simulink model "tesdd"  (R2012b)
settings: Solver=ode45  StartTime=0.0  StopTime=25000  RelTol=1e-3
undefined symbols (not defined in the file or in its folder): pfb_coeff_gen_calc, sfp
undefined symbols (not defined in the file): SL, transtable
libraries: xbsIndex_r4 x5296, casper_library_misc x104, casper_library_delays x24, xps_library x14, maddogLibrary x4, simulink x2
(part 37 of 52)

== system tesdd/FRD2/DFT/costable/mem ==
  note: Undo data manipulation on way in and redo on way out for simulated data
  note: Undo address
      | manipulation for
      | simulated data
  In1 : Inport
  In2 : Inport  Port=2
  In3 : Inport  Port=3
  Disregard Subsystem : xbsIndex_r4/Disregard Subsystem  Tag=discardX  block_type=disregard
  calc_add : Subsystem  mask{data_width=16, addr_width=11, sample_rate=sample_rate}
      mask prompts: data_width "data width"; addr_width "address width"; sample_rate "sample rate"
  ram : xbsIndex_r4/Single Port RAM  depth=2^addr_width  initVector=init_vals  distributed_mem=Block RAM  write_mode=Read After Write  rst=off  init_reg=0  en=off  latency=1  dbl_ovrd=off  optimize=Area  block_type=spram
  sim_addr : xbsIndex_r4/Gateway In  gui_display_data_type=Fixed-point  arith_type=Unsigned  n_bits=addr_width  bin_pt=0  preci_type=Single  exp_width=8  frac_width=24  quantization=Truncate  overflow=Wrap  period=sample_rate  dbl_ovrd=off  timing_constraint=None  locs_specified=off  LOCs={}  UseAsADC=off  ADCChannel='1'  inherit_from_input=off  hdl_port=on  block_type=gatewayin
      settings: infoedit="Gateway in block.  Converts inputs of type Simulink integer, double and fixed point to  Xilinx fixed point type.<br><br>Hardware notes:  In hardware these blocks become top level input ports."  xl_area=[0, 0, 0, 0, 0, 0, 0]  sginterface={'Nallatech'=>{'xdspkit'=>{'non_memory_mapped_port'=>'sim_addr'}},'Xilinx'=>{'jtaghwcosim'=>{'non_memory_mapped_port'=>'sim_addr'},'xdspkit'=>{'non_memory_mapped_port'=>'sim_addr'}}}
  sim_data_in : xbsIndex_r4/Gateway In  gui_display_data_type=Fixed-point  arith_type=Unsigned  n_bits=16  bin_pt=14  preci_type=Single  exp_width=8  frac_width=24  quantization=Truncate  overflow=Wrap  period=sample_rate  dbl_ovrd=off  timing_constraint=None  locs_specified=off  LOCs={}  UseAsADC=off  ADCChannel='1'  inherit_from_input=off  hdl_port=on  block_type=gatewayin
      settings: xl_area=[0, 0, 0, 0, 0, 0, 0]  sginterface={'Nallatech'=>{'xdspkit'=>{'non_memory_mapped_port'=>'sim_data_in'}},'Xilinx'=>{'jtaghwcosim'=>{'non_memory_mapped_port'=>'sim_data_in'},'xdspkit'=>{'non_memory_mapped_port'=>'sim_data_in'}}}
  sim_data_out : xbsIndex_r4/Gateway Out  inherit_from_input=off  hdl_port=on  timing_constraint=None  locs_specified=off  LOCs={'B21','B22','A22','B23','B19','C19','A20','A21','A23','B24','A24','A25','E18','D18','C18','B18'}  UseAsDAC=off  DACChannel='1'  block_type=gatewayout
      settings: infoedit="Gateway out block.  Converts Xilinx fixed point inputs into ouputs of type Simulink integer, double, or fixed point.<P><P>Hardware notes:  In hardware these blocks become top level output ports or are discarded, depending on how they are configured."  xl_area=[0, 0, 0, 0, 0, 0, 0]  sginterface={'Nallatech'=>{'xdspkit'=>{'non_memory_mapped_port'=>'sim_data_out'}},'Xilinx'=>{'jtaghwcosim'=>{'non_memory_mapped_port'=>'sim_data_out'},'xdspkit'=>{'non_memory_mapped_port'=>'sim_data_out'}}}
  sim_munge_in : Subsystem  AncestorBlock=casper_library_flow_control/munge  mask(munge){divisions=1, div_size=16, order=[0], arith_type_out=Signed  (2's comp), bin_pt_out=14}
      mask prompts: divisions "Number of divisions"; div_size "Division size (bits)"; order "Division packing order"; arith_type_out "Output arithmetic type"; bin_pt_out "Output binary point"
      mask help: Splits an input bus into the specified number of divisions and then recombines them in the order specified (most significant division = 0,least = number divisions-1)
      mask init:
      | munge_init(gcb, ...
      |     'divisions', divisions, ...
      |     'div_size', div_size, ...
      |     'order', order, ...
      |     'arith_type_out', arith_type_out, ...
      |     'bin_pt_out', bin_pt_out);
      settings: AttributesFormatString=|
      | split:16
      | join:0
      | Signed  (2's comp) [16,14]
      mask TypeOptions arith_type_out: Unsigned | Signed  (2's comp) | Floating-point
  sim_munge_out : Subsystem  AncestorBlock=casper_library_flow_control/munge  mask(munge){divisions=1, div_size=16, order=[0], arith_type_out=Unsigned, bin_pt_out=14}
      mask prompts: divisions "Number of divisions"; div_size "Division size (bits)"; order "Division packing order"; arith_type_out "Output arithmetic type"; bin_pt_out "Output binary point"
      mask help: Splits an input bus into the specified number of divisions and then recombines them in the order specified (most significant division = 0,least = number divisions-1)
      mask init:
      | munge_init(gcb, ...
      |     'divisions', divisions, ...
      |     'div_size', div_size, ...
      |     'order', order, ...
      |     'arith_type_out', arith_type_out, ...
      |     'bin_pt_out', bin_pt_out);
      settings: AttributesFormatString=|
      | split:16
      | join:0
      | Unsigned [16,14]
      mask TypeOptions arith_type_out: Unsigned | Signed  (2's comp) | Floating-point
  sim_we : xbsIndex_r4/Gateway In  gui_display_data_type=Fixed-point  arith_type=Boolean  n_bits=1  bin_pt=0  preci_type=Single  exp_width=8  frac_width=24  quantization=Truncate  overflow=Wrap  period=sample_rate  dbl_ovrd=off  timing_constraint=None  locs_specified=off  LOCs={}  UseAsADC=off  ADCChannel='1'  inherit_from_input=off  hdl_port=on  block_type=gatewayin
      settings: infoedit="Gateway in block.  Converts inputs of type Simulink integer, double and fixed point to  Xilinx fixed point type.<br><br>Hardware notes:  In hardware these blocks become top level input ports."  xl_area=[0, 0, 0, 0, 0, 0, 0]  sginterface={'Nallatech'=>{'xdspkit'=>{'non_memory_mapped_port'=>'sim_we'}},'Xilinx'=>{'jtaghwcosim'=>{'non_memory_mapped_port'=>'sim_we'},'xdspkit'=>{'non_memory_mapped_port'=>'sim_we'}}}
  Out1 : Outport
  wires:
  calc_add/1(out) -> ram/1
  sim_munge_out/1(dout) -> sim_data_out/1
  In1/1 -> sim_addr/1
  In2/1 -> sim_data_in/1
  sim_data_out/1 -> Out1/1
  In3/1 -> sim_we/1
  sim_addr/1 -> calc_add/1(in)
  sim_data_in/1 -> sim_munge_in/1(din)
  sim_we/1 -> ram/3
  ram/1 -> sim_munge_out/1(din)
  sim_munge_in/1(dout) -> ram/2

== system tesdd/FRD2/DFT/costable/munge_in ==
  din : Inport
  reinterpret_out : xbsIndex_r4/Reinterpret  force_arith_type=on  arith_type=Unsigned  force_bin_pt=on  bin_pt=14  block_type=reinterpret
  dout : Outport
  wires:
  reinterpret_out/1 -> dout/1
  din/1 -> reinterpret_out/1

== system tesdd/FRD2/DFT/costable/munge_out ==
  din : Inport
  reinterpret_out : xbsIndex_r4/Reinterpret  force_arith_type=on  arith_type="Signed  (2's comp)"  force_bin_pt=on  bin_pt=14  block_type=reinterpret
  dout : Outport
  wires:
  reinterpret_out/1 -> dout/1
  din/1 -> reinterpret_out/1

== system tesdd/FRD2/DFT/sintable/calc_add ==
  note: Use behavioural HDL
      | so that gets optimised
      | to minimum logic
  note: If reading/writing words
      | smaller than 32 bits,
      | change address so
      | that addressing is
      | big endian instead of
      | little, otherwise
      | pass through
  in : Inport
  add_sub : xbsIndex_r4/AddSub  mode=Subtraction  use_carryin=off  use_carryout=off  en=off  latency=0  precision=User Defined  arith_type=Unsigned  n_bits=max(1, log2(32/data_width))  bin_pt=0  quantization=Truncate  overflow=Wrap  dbl_ovrd=off  use_behavioral_HDL=on  hw_selection=Fabric  pipelined=off  block_type=addsub
  concat : xbsIndex_r4/Concat  num_inputs=2  dbl_ovrd=off  block_type=concat
  const : xbsIndex_r4/Constant  const=max(0, 32/data_width-1)  gui_display_data_type=Fixed-point  arith_type=Unsigned  n_bits=max(1, log2(32/data_width))  bin_pt=0  preci_type=Single  exp_width=8  frac_width=24  explicit_period=on  period=sample_rate  equ=P=C  opselect=C  inp2=PCIN>>17  opr=+  inp1=P  carry=CIN  dbl_ovrd=off  block_type=constant
      settings: block_version=11.4
  convert_addr : xbsIndex_r4/Convert  gui_display_data_type=Fixed-point  arith_type=Unsigned  n_bits=addr_width  bin_pt=0  float_type=Single  exp_bits=8  fraction_bits=24  quantization=Truncate  overflow=Wrap  en=off  latency=0  dbl_ovrd=off  pipeline=off  block_type=convert
      settings: xl_area=[0, 0, 0, 0, 0, 0, 0]
  lsw : xbsIndex_r4/Slice  nbits=max(1, log2(32/data_width))  boolean_output=off  mode=Lower Bit Location + Width  bit1=0  base1=MSB of Input  bit0=0  base0=LSB of Input  dbl_ovrd=off  block_type=slice
  manipulate : xbsIndex_r4/Constant  const=min(1, floor(32/data_width) - 1)  gui_display_data_type=Fixed-point  arith_type=Unsigned  n_bits=1  bin_pt=0  preci_type=Single  exp_width=8  frac_width=24  explicit_period=on  period=sample_rate  equ=P=C  opselect=C  inp2=PCIN>>17  opr=+  inp1=P  carry=CIN  dbl_ovrd=off  block_type=constant
      settings: block_version=11.4
  msw : xbsIndex_r4/Slice  nbits=addr_width - max(1, log2(32/data_width))  boolean_output=off  mode=Upper Bit Location + Width  bit1=0  base1=MSB of Input  bit0=0  base0=LSB of Input  dbl_ovrd=off  block_type=slice
  mux : xbsIndex_r4/Mux  inputs=2  en=off  latency=0  precision=Full  arith_type=Unsigned  n_bits=16  bin_pt=14  quantization=Truncate  overflow=Wrap  dbl_ovrd=off  block_type=mux
      settings: block_version=11.4
  out : Outport
  wires:
  convert_addr/1 -> mux/2, msw/1, lsw/1
  const/1 -> add_sub/1
  lsw/1 -> add_sub/2
  mux/1 -> out/1
  manipulate/1 -> mux/1
  concat/1 -> mux/3
  msw/1 -> concat/1
  add_sub/1 -> concat/2
  in/1 -> convert_addr/1

== system tesdd/FRD2/DFT/sintable/mem ==
  note: Undo data manipulation on way in and redo on way out for simulated data
  note: Undo address
      | manipulation for
      | simulated data
  In1 : Inport
  In2 : Inport  Port=2
  In3 : Inport  Port=3
  Disregard Subsystem : xbsIndex_r4/Disregard Subsystem  Tag=discardX  block_type=disregard
  calc_add : Subsystem  mask{data_width=16, addr_width=11, sample_rate=sample_rate}
      mask prompts: data_width "data width"; addr_width "address width"; sample_rate "sample rate"
  ram : xbsIndex_r4/Single Port RAM  depth=2^addr_width  initVector=init_vals  distributed_mem=Block RAM  write_mode=Read After Write  rst=off  init_reg=0  en=off  latency=1  dbl_ovrd=off  optimize=Area  block_type=spram
  sim_addr : xbsIndex_r4/Gateway In  gui_display_data_type=Fixed-point  arith_type=Unsigned  n_bits=addr_width  bin_pt=0  preci_type=Single  exp_width=8  frac_width=24  quantization=Truncate  overflow=Wrap  period=sample_rate  dbl_ovrd=off  timing_constraint=None  locs_specified=off  LOCs={}  UseAsADC=off  ADCChannel='1'  inherit_from_input=off  hdl_port=on  block_type=gatewayin
      settings: infoedit="Gateway in block.  Converts inputs of type Simulink integer, double and fixed point to  Xilinx fixed point type.<br><br>Hardware notes:  In hardware these blocks become top level input ports."  xl_area=[0, 0, 0, 0, 0, 0, 0]  sginterface={'Nallatech'=>{'xdspkit'=>{'non_memory_mapped_port'=>'sim_addr'}},'Xilinx'=>{'jtaghwcosim'=>{'non_memory_mapped_port'=>'sim_addr'},'xdspkit'=>{'non_memory_mapped_port'=>'sim_addr'}}}
  sim_data_in : xbsIndex_r4/Gateway In  gui_display_data_type=Fixed-point  arith_type=Unsigned  n_bits=16  bin_pt=14  preci_type=Single  exp_width=8  frac_width=24  quantization=Truncate  overflow=Wrap  period=sample_rate  dbl_ovrd=off  timing_constraint=None  locs_specified=off  LOCs={}  UseAsADC=off  ADCChannel='1'  inherit_from_input=off  hdl_port=on  block_type=gatewayin
      settings: xl_area=[0, 0, 0, 0, 0, 0, 0]  sginterface={'Nallatech'=>{'xdspkit'=>{'non_memory_mapped_port'=>'sim_data_in'}},'Xilinx'=>{'jtaghwcosim'=>{'non_memory_mapped_port'=>'sim_data_in'},'xdspkit'=>{'non_memory_mapped_port'=>'sim_data_in'}}}
  sim_data_out : xbsIndex_r4/Gateway Out  inherit_from_input=off  hdl_port=on  timing_constraint=None  locs_specified=off  LOCs={'B21','B22','A22','B23','B19','C19','A20','A21','A23','B24','A24','A25','E18','D18','C18','B18'}  UseAsDAC=off  DACChannel='1'  block_type=gatewayout
      settings: infoedit="Gateway out block.  Converts Xilinx fixed point inputs into ouputs of type Simulink integer, double, or fixed point.<P><P>Hardware notes:  In hardware these blocks become top level output ports or are discarded, depending on how they are configured."  xl_area=[0, 0, 0, 0, 0, 0, 0]  sginterface={'Nallatech'=>{'xdspkit'=>{'non_memory_mapped_port'=>'sim_data_out'}},'Xilinx'=>{'jtaghwcosim'=>{'non_memory_mapped_port'=>'sim_data_out'},'xdspkit'=>{'non_memory_mapped_port'=>'sim_data_out'}}}
  sim_munge_in : Subsystem  AncestorBlock=casper_library_flow_control/munge  mask(munge){divisions=1, div_size=16, order=[0], arith_type_out=Signed  (2's comp), bin_pt_out=14}
      mask prompts: divisions "Number of divisions"; div_size "Division size (bits)"; order "Division packing order"; arith_type_out "Output arithmetic type"; bin_pt_out "Output binary point"
      mask help: Splits an input bus into the specified number of divisions and then recombines them in the order specified (most significant division = 0,least = number divisions-1)
      mask init:
      | munge_init(gcb, ...
      |     'divisions', divisions, ...
      |     'div_size', div_size, ...
      |     'order', order, ...
      |     'arith_type_out', arith_type_out, ...
      |     'bin_pt_out', bin_pt_out);
      settings: AttributesFormatString=|
      | split:16
      | join:0
      | Signed  (2's comp) [16,14]
      mask TypeOptions arith_type_out: Unsigned | Signed  (2's comp) | Floating-point
  sim_munge_out : Subsystem  AncestorBlock=casper_library_flow_control/munge  mask(munge){divisions=1, div_size=16, order=[0], arith_type_out=Unsigned, bin_pt_out=14}
      mask prompts: divisions "Number of divisions"; div_size "Division size (bits)"; order "Division packing order"; arith_type_out "Output arithmetic type"; bin_pt_out "Output binary point"
      mask help: Splits an input bus into the specified number of divisions and then recombines them in the order specified (most significant division = 0,least = number divisions-1)
      mask init:
      | munge_init(gcb, ...
      |     'divisions', divisions, ...
      |     'div_size', div_size, ...
      |     'order', order, ...
      |     'arith_type_out', arith_type_out, ...
      |     'bin_pt_out', bin_pt_out);
      settings: AttributesFormatString=|
      | split:16
      | join:0
      | Unsigned [16,14]
      mask TypeOptions arith_type_out: Unsigned | Signed  (2's comp) | Floating-point
  sim_we : xbsIndex_r4/Gateway In  gui_display_data_type=Fixed-point  arith_type=Boolean  n_bits=1  bin_pt=0  preci_type=Single  exp_width=8  frac_width=24  quantization=Truncate  overflow=Wrap  period=sample_rate  dbl_ovrd=off  timing_constraint=None  locs_specified=off  LOCs={}  UseAsADC=off  ADCChannel='1'  inherit_from_input=off  hdl_port=on  block_type=gatewayin
      settings: infoedit="Gateway in block.  Converts inputs of type Simulink integer, double and fixed point to  Xilinx fixed point type.<br><br>Hardware notes:  In hardware these blocks become top level input ports."  xl_area=[0, 0, 0, 0, 0, 0, 0]  sginterface={'Nallatech'=>{'xdspkit'=>{'non_memory_mapped_port'=>'sim_we'}},'Xilinx'=>{'jtaghwcosim'=>{'non_memory_mapped_port'=>'sim_we'},'xdspkit'=>{'non_memory_mapped_port'=>'sim_we'}}}
  Out1 : Outport
  wires:
  calc_add/1(out) -> ram/1
  sim_munge_out/1(dout) -> sim_data_out/1
  In1/1 -> sim_addr/1
  In2/1 -> sim_data_in/1
  sim_data_out/1 -> Out1/1
  In3/1 -> sim_we/1
  sim_addr/1 -> calc_add/1(in)
  sim_data_in/1 -> sim_munge_in/1(din)
  sim_we/1 -> ram/3
  ram/1 -> sim_munge_out/1(din)
  sim_munge_in/1(dout) -> ram/2

== system tesdd/FRD2/DFT/sintable/munge_in ==
  din : Inport
  reinterpret_out : xbsIndex_r4/Reinterpret  force_arith_type=on  arith_type=Unsigned  force_bin_pt=on  bin_pt=14  block_type=reinterpret
  dout : Outport
  wires:
  reinterpret_out/1 -> dout/1
  din/1 -> reinterpret_out/1

== system tesdd/FRD2/DFT/sintable/munge_out ==
  din : Inport
  reinterpret_out : xbsIndex_r4/Reinterpret  force_arith_type=on  arith_type="Signed  (2's comp)"  force_bin_pt=on  bin_pt=14  block_type=reinterpret
  dout : Outport
  wires:
  reinterpret_out/1 -> dout/1
  din/1 -> reinterpret_out/1

== system tesdd/FRD2/trIQ/tr/calc_add ==
  note: Use behavioural HDL
      | so that gets optimised
      | to minimum logic
  note: If reading/writing words
      | smaller than 32 bits,
      | change address so
      | that addressing is
      | big endian instead of
      | little, otherwise
      | pass through
  in : Inport
  add_sub : xbsIndex_r4/AddSub  mode=Subtraction  use_carryin=off  use_carryout=off  en=off  latency=0  precision=User Defined  arith_type=Unsigned  n_bits=max(1, log2(32/data_width))  bin_pt=0  quantization=Truncate  overflow=Wrap  dbl_ovrd=off  use_behavioral_HDL=on  hw_selection=Fabric  pipelined=off  block_type=addsub
  concat : xbsIndex_r4/Concat  num_inputs=2  dbl_ovrd=off  block_type=concat
  const : xbsIndex_r4/Constant  const=max(0, 32/data_width-1)  gui_display_data_type=Fixed-point  arith_type=Unsigned  n_bits=max(1, log2(32/data_width))  bin_pt=0  preci_type=Single  exp_width=8  frac_width=24  explicit_period=on  period=sample_rate  equ=P=C  opselect=C  inp2=PCIN>>17  opr=+  inp1=P  carry=CIN  dbl_ovrd=off  block_type=constant
      settings: block_version=11.4
  convert_addr : xbsIndex_r4/Convert  gui_display_data_type=Fixed-point  arith_type=Unsigned  n_bits=addr_width  bin_pt=0  float_type=Single  exp_bits=8  fraction_bits=24  quantization=Truncate  overflow=Wrap  en=off  latency=0  dbl_ovrd=off  pipeline=off  block_type=convert
      settings: xl_area=[0, 0, 0, 0, 0, 0, 0]
  lsw : xbsIndex_r4/Slice  nbits=max(1, log2(32/data_width))  boolean_output=off  mode=Lower Bit Location + Width  bit1=0  base1=MSB of Input  bit0=0  base0=LSB of Input  dbl_ovrd=off  block_type=slice
  manipulate : xbsIndex_r4/Constant  const=min(1, floor(32/data_width) - 1)  gui_display_data_type=Fixed-point  arith_type=Unsigned  n_bits=1  bin_pt=0  preci_type=Single  exp_width=8  frac_width=24  explicit_period=on  period=sample_rate  equ=P=C  opselect=C  inp2=PCIN>>17  opr=+  inp1=P  carry=CIN  dbl_ovrd=off  block_type=constant
      settings: block_version=11.4
  msw : xbsIndex_r4/Slice  nbits=addr_width - max(1, log2(32/data_width))  boolean_output=off  mode=Upper Bit Location + Width  bit1=0  base1=MSB of Input  bit0=0  base0=LSB of Input  dbl_ovrd=off  block_type=slice
  mux : xbsIndex_r4/Mux  inputs=2  en=off  latency=0  precision=Full  arith_type=Unsigned  n_bits=16  bin_pt=14  quantization=Truncate  overflow=Wrap  dbl_ovrd=off  block_type=mux
      settings: block_version=11.4
  out : Outport
  wires:
  convert_addr/1 -> mux/2, msw/1, lsw/1
  const/1 -> add_sub/1
  lsw/1 -> add_sub/2
  mux/1 -> out/1
  manipulate/1 -> mux/1
  concat/1 -> mux/3
  msw/1 -> concat/1
  add_sub/1 -> concat/2
  in/1 -> convert_addr/1

== system tesdd/FRD2/trIQ/tr/mem ==
  note: Undo data manipulation on way in and redo on way out for simulated data
  note: Undo address
      | manipulation for
      | simulated data
  In1 : Inport
  In2 : Inport  Port=2
  In3 : Inport  Port=3
  Disregard Subsystem : xbsIndex_r4/Disregard Subsystem  Tag=discardX  block_type=disregard
  calc_add : Subsystem  mask{data_width=32, addr_width=10, sample_rate=sample_rate}
      mask prompts: data_width "data width"; addr_width "address width"; sample_rate "sample rate"
  ram : xbsIndex_r4/Single Port RAM  depth=2^addr_width  initVector=init_vals  distributed_mem=Block RAM  write_mode=Read After Write  rst=off  init_reg=0  en=off  latency=1  dbl_ovrd=off  optimize=Area  block_type=spram
  sim_addr : xbsIndex_r4/Gateway In  gui_display_data_type=Fixed-point  arith_type=Unsigned  n_bits=addr_width  bin_pt=0  preci_type=Single  exp_width=8  frac_width=24  quantization=Truncate  overflow=Wrap  period=sample_rate  dbl_ovrd=off  timing_constraint=None  locs_specified=off  LOCs={}  UseAsADC=off  ADCChannel='1'  inherit_from_input=off  hdl_port=on  block_type=gatewayin
      settings: infoedit="Gateway in block.  Converts inputs of type Simulink integer, double and fixed point to  Xilinx fixed point type.<br><br>Hardware notes:  In hardware these blocks become top level input ports."  xl_area=[0, 0, 0, 0, 0, 0, 0]  sginterface={'Nallatech'=>{'xdspkit'=>{'non_memory_mapped_port'=>'sim_addr'}},'Xilinx'=>{'jtaghwcosim'=>{'non_memory_mapped_port'=>'sim_addr'},'xdspkit'=>{'non_memory_mapped_port'=>'sim_addr'}}}
  sim_data_in : xbsIndex_r4/Gateway In  gui_display_data_type=Fixed-point  arith_type=Unsigned  n_bits=32  bin_pt=0  preci_type=Single  exp_width=8  frac_width=24  quantization=Truncate  overflow=Wrap  period=sample_rate  dbl_ovrd=off  timing_constraint=None  locs_specified=off  LOCs={}  UseAsADC=off  ADCChannel='1'  inherit_from_input=off  hdl_port=on  block_type=gatewayin
      settings: xl_area=[0, 0, 0, 0, 0, 0, 0]  sginterface={'Nallatech'=>{'xdspkit'=>{'non_memory_mapped_port'=>'sim_data_in'}},'Xilinx'=>{'jtaghwcosim'=>{'non_memory_mapped_port'=>'sim_data_in'},'xdspkit'=>{'non_memory_mapped_port'=>'sim_data_in'}}}
  sim_data_out : xbsIndex_r4/Gateway Out  inherit_from_input=off  hdl_port=on  timing_constraint=None  locs_specified=off  LOCs={'B21','B22','A22','B23','B19','C19','A20','A21','A23','B24','A24','A25','E18','D18','C18','B18'}  UseAsDAC=off  DACChannel='1'  block_type=gatewayout
      settings: infoedit="Gateway out block.  Converts Xilinx fixed point inputs into ouputs of type Simulink integer, double, or fixed point.<P><P>Hardware notes:  In hardware these blocks become top level output ports or are discarded, depending on how they are configured."  xl_area=[0, 0, 0, 0, 0, 0, 0]  sginterface={'Nallatech'=>{'xdspkit'=>{'non_memory_mapped_port'=>'sim_data_out'}},'Xilinx'=>{'jtaghwcosim'=>{'non_memory_mapped_port'=>'sim_data_out'},'xdspkit'=>{'non_memory_mapped_port'=>'sim_data_out'}}}
  sim_munge_in : Subsystem  AncestorBlock=casper_library_flow_control/munge  mask(munge){divisions=1, div_size=32, order=[0], arith_type_out=Unsigned, bin_pt_out=0}
      mask prompts: divisions "Number of divisions"; div_size "Division size (bits)"; order "Division packing order"; arith_type_out "Output arithmetic type"; bin_pt_out "Output binary point"
      mask help: Splits an input bus into the specified number of divisions and then recombines them in the order specified (most significant division = 0,least = number divisions-1)
      mask init:
      | munge_init(gcb, ...
      |     'divisions', divisions, ...
      |     'div_size', div_size, ...
      |     'order', order, ...
      |     'arith_type_out', arith_type_out, ...
      |     'bin_pt_out', bin_pt_out);
      settings: AttributesFormatString=|
      | split:32
      | join:0
      | Unsigned [32,0]
      mask TypeOptions arith_type_out: Unsigned | Signed  (2's comp) | Floating-point
  sim_munge_out : Subsystem  AncestorBlock=casper_library_flow_control/munge  mask(munge){divisions=1, div_size=32, order=[0], arith_type_out=Unsigned, bin_pt_out=0}
      mask prompts: divisions "Number of divisions"; div_size "Division size (bits)"; order "Division packing order"; arith_type_out "Output arithmetic type"; bin_pt_out "Output binary point"
      mask help: Splits an input bus into the specified number of divisions and then recombines them in the order specified (most significant division = 0,least = number divisions-1)
      mask init:
      | munge_init(gcb, ...
      |     'divisions', divisions, ...
      |     'div_size', div_size, ...
      |     'order', order, ...
      |     'arith_type_out', arith_type_out, ...
      |     'bin_pt_out', bin_pt_out);
      settings: AttributesFormatString=|
      | split:32
      | join:0
      | Unsigned [32,0]
      mask TypeOptions arith_type_out: Unsigned | Signed  (2's comp) | Floating-point
  sim_we : xbsIndex_r4/Gateway In  gui_display_data_type=Fixed-point  arith_type=Boolean  n_bits=1  bin_pt=0  preci_type=Single  exp_width=8  frac_width=24  quantization=Truncate  overflow=Wrap  period=sample_rate  dbl_ovrd=off  timing_constraint=None  locs_specified=off  LOCs={}  UseAsADC=off  ADCChannel='1'  inherit_from_input=off  hdl_port=on  block_type=gatewayin
      settings: infoedit="Gateway in block.  Converts inputs of type Simulink integer, double and fixed point to  Xilinx fixed point type.<br><br>Hardware notes:  In hardware these blocks become top level input ports."  xl_area=[0, 0, 0, 0, 0, 0, 0]  sginterface={'Nallatech'=>{'xdspkit'=>{'non_memory_mapped_port'=>'sim_we'}},'Xilinx'=>{'jtaghwcosim'=>{'non_memory_mapped_port'=>'sim_we'},'xdspkit'=>{'non_memory_mapped_port'=>'sim_we'}}}
  Out1 : Outport
  wires:
  calc_add/1(out) -> ram/1
  sim_munge_out/1(dout) -> sim_data_out/1
  In1/1 -> sim_addr/1
  In2/1 -> sim_data_in/1
  sim_data_out/1 -> Out1/1
  In3/1 -> sim_we/1
  sim_addr/1 -> calc_add/1(in)
  sim_data_in/1 -> sim_munge_in/1(din)
  sim_we/1 -> ram/3
  ram/1 -> sim_munge_out/1(din)
  sim_munge_in/1(dout) -> ram/2

== system tesdd/FRD2/trIQ/tr/munge_in ==
  din : Inport
  reinterpret_out : xbsIndex_r4/Reinterpret  force_arith_type=on  arith_type=Unsigned  force_bin_pt=on  bin_pt=0  block_type=reinterpret
  dout : Outport
  wires:
  reinterpret_out/1 -> dout/1
  din/1 -> reinterpret_out/1

== system tesdd/FRD2/trIQ/tr/munge_out ==
  din : Inport
  reinterpret_out : xbsIndex_r4/Reinterpret  force_arith_type=on  arith_type=Unsigned  force_bin_pt=on  bin_pt=0  block_type=reinterpret
  dout : Outport
  wires:
  reinterpret_out/1 -> dout/1
  din/1 -> reinterpret_out/1

== system tesdd/WindowAndFFT/FFT512_/FFT_DIT512_/Butterfly ==
  note: same delay as cmpkx mult
  ImInOne : Inport
  ReInOne : Inport  Port=2
  ImInTw : Inport  Port=3
  ReInTw : Inport  Port=4
  TwIm : Inport  Port=5
  TwRe : Inport  Port=6
  dvld : Inport  Port=7
  syncin : Inport  Port=8
  AddSub : xbsIndex_r4/AddSub  mode=Addition  use_carryin=off  use_carryout=off  en=off  latency=1  precision=Full  arith_type=Unsigned  n_bits=16  bin_pt=14  quantization=Truncate  overflow=Wrap  dbl_ovrd=off  use_behavioral_HDL=off  hw_selection=Fabric  pipelined=off  block_type=addsub
  AddSub1 : xbsIndex_r4/AddSub  mode=Addition  use_carryin=off  use_carryout=off  en=off  latency=1  precision=Full  arith_type=Unsigned  n_bits=16  bin_pt=14  quantization=Truncate  overflow=Wrap  dbl_ovrd=off  use_behavioral_HDL=off  hw_selection=Fabric  pipelined=off  block_type=addsub
  "Complex Multiplier 5.0 " : xbsIndex_r4/Complex Multiplier 5.0   hasatlast=on  hasatuser=off  atuserwidth=1  hasbtlast=off  hasbtuser=off  btuserwidth=1  multtype=Use_Mults  optimizegoal=Resources  flowcontrol=NonBlocking  outputwidth=33  roundmode=Truncate  hasctrltlast=off  hasctrltuser=off  ctrltuserwidth=1  outtlastbehv=Pass_A_TLAST  latencyconfig=Automatic  minimumlatency=37  aclken=off  aresetn=off  trim_axipin_name=on  aportwidth=63  bportwidth=63  ip_name=Complex Multiplier  ip_version=5.0  dsptool_ready=true  ipcore_usecache=true  ipcore_useipmodelcache=true  ipcore_verbose=false  ipcore_latency_parameter='minimumlatency'  wrapper_available=true  port_translation_map={ 'aclken' => 'en', 'aresetn' => 'rst'}  structural_sim=false  block_type=cmpy_v5_0
  Complex to Magnitude-Angle{,1..5} (6 alike) : ComplexToMagnitudeAngle
  Convert{,1..7} (8 alike) : xbsIndex_r4/Convert  gui_display_data_type=Fixed-point  arith_type="Signed  (2's comp)"  n_bits=16  bin_pt=14  float_type=Single  exp_bits=8  fraction_bits=24  quantization=Truncate  overflow=Wrap  en=off  latency=0  dbl_ovrd=off  pipeline=off  block_type=convert
  Delay : xbsIndex_r4/Delay  rst=off  infoeditControl=Selection of Reset will increase slice count due to use of real FFs and instead of SRLs  en=off  latency=6  dbl_ovrd=off  reg_retiming=off  block_type=delay
  Delay1 : xbsIndex_r4/Delay  rst=off  infoeditControl=Selection of Reset will increase slice count due to use of real FFs and instead of SRLs  en=off  latency=6  dbl_ovrd=off  reg_retiming=off  block_type=delay
  Delay2 : xbsIndex_r4/Delay  rst=off  infoeditControl=Selection of Reset will increase slice count due to use of real FFs and instead of SRLs  en=off  latency=1  dbl_ovrd=off  reg_retiming=off  block_type=delay
  Delay3 : xbsIndex_r4/Delay  rst=off  infoeditControl=Selection of Reset will increase slice count due to use of real FFs and instead of SRLs  en=off  latency=1  dbl_ovrd=off  reg_retiming=off  block_type=delay
  Gateway Out{1..14} (14 alike) : xbsIndex_r4/Gateway Out  inherit_from_input=off  hdl_port=on  timing_constraint=None  locs_specified=off  LOCs={}  UseAsDAC=off  DACChannel='1'  block_type=gatewayout
  Real-Imag to Complex{,1..5} (6 alike) : RealImagToComplex
  buttscope : Scope  NumInputPorts=6
      settings: YMin=-5~-5~-5~-5~-5~-5  YMax=5~5~5~5~5~5  SaveName=ScopeData4
  buttscope1 : Scope  NumInputPorts=8
      settings: YMin=-5~-5~-5~-5~-5~-5~-5~-5  YMax=5~5~5~5~5~5~5~5  SaveName=ScopeData6
  Imut : Outport
  ReOut : Outport  Port=2
  dvldout : Outport  Port=3
  syncout : Outport  Port=4
  wires:
  ReInOne/1 -> Convert7/1
  ImInOne/1 -> Convert6/1
  AddSub/1 -> Gateway Out6/1, Imut/1
  AddSub1/1 -> Gateway Out2/1, ReOut/1
  ImInTw/1 -> Convert3/1
  ReInTw/1 -> Convert2/1
  Delay/1 -> Gateway Out7/1, AddSub/1
  Delay1/1 -> Gateway Out3/1, AddSub1/1
  TwIm/1 -> Convert4/1
  TwRe/1 -> Convert5/1
  dvld/1 -> "Complex Multiplier 5.0 "/5, "Complex Multiplier 5.0 "/1
  Convert6/1 -> Delay/1
  Convert7/1 -> Delay1/1
  Convert3/1 -> "Complex Multiplier 5.0 "/3, Gateway Out11/1
  Convert2/1 -> "Complex Multiplier 5.0 "/4, Gateway Out12/1
  Convert4/1 -> "Complex Multiplier 5.0 "/6, Gateway Out5/1
  Convert5/1 -> "Complex Multiplier 5.0 "/7, Gateway Out8/1
  Convert1/1 -> Gateway Out10/1, Gateway Out4/1, AddSub1/2
  syncin/1 -> Gateway Out14/1, "Complex Multiplier 5.0 "/2
  "Complex Multiplier 5.0 "/4 -> Convert1/1
  "Complex Multiplier 5.0 "/3 -> Convert/1
  "Complex Multiplier 5.0 "/1 -> Delay2/1
  "Complex Multiplier 5.0 "/2 -> Gateway Out13/1, Delay3/1
  Convert/1 -> Gateway Out9/1, Gateway Out1/1, AddSub/2
  Delay2/1 -> dvldout/1
  Delay3/1 -> syncout/1
  Real-Imag to Complex/1 -> Complex to Magnitude-Angle/1
  Real-Imag to Complex1/1 -> Complex to Magnitude-Angle1/1
  Real-Imag to Complex2/1 -> Complex to Magnitude-Angle2/1
  Complex to Magnitude-Angle/1 -> buttscope1/1
  Complex to Magnitude-Angle/2 -> buttscope1/2
  Complex to Magnitude-Angle1/1 -> buttscope1/3
  Complex to Magnitude-Angle1/2 -> buttscope1/4
  Complex to Magnitude-Angle2/1 -> buttscope1/5
  Complex to Magnitude-Angle2/2 -> buttscope1/6
  Gateway Out11/1 -> Real-Imag to Complex/2
  Gateway Out12/1 -> Real-Imag to Complex/1
  Gateway Out5/1 -> Real-Imag to Complex1/2
  Gateway Out8/1 -> Real-Imag to Complex1/1
  Gateway Out9/1 -> Real-Imag to Complex2/2
  Gateway Out10/1 -> Real-Imag to Complex2/1
  Gateway Out13/1 -> buttscope1/7
  Gateway Out14/1 -> buttscope1/8
  Real-Imag to Complex3/1 -> Complex to Magnitude-Angle3/1
  Real-Imag to Complex4/1 -> Complex to Magnitude-Angle4/1
  Real-Imag to Complex5/1 -> Complex to Magnitude-Angle5/1
  Gateway Out7/1 -> Real-Imag to Complex3/2
  Gateway Out3/1 -> Real-Imag to Complex3/1
  Complex to Magnitude-Angle3/1 -> buttscope/1
  Complex to Magnitude-Angle3/2 -> buttscope/2
  Gateway Out1/1 -> Real-Imag to Complex4/2
  Gateway Out4/1 -> Real-Imag to Complex4/1
  Complex to Magnitude-Angle4/1 -> buttscope/3
  Complex to Magnitude-Angle4/2 -> buttscope/4
  Gateway Out6/1 -> Real-Imag to Complex5/2
  Gateway Out2/1 -> Real-Imag to Complex5/1
  Complex to Magnitude-Angle5/1 -> buttscope/5
  Complex to Magnitude-Angle5/2 -> buttscope/6

== system tesdd/WindowAndFFT/FFT512_/FFT_DIT512_/Butterfly1 ==
  note: same delay as cmpkx mult
  ImInOne : Inport
  ReInOne : Inport  Port=2
  ImInTw : Inport  Port=3
  ReInTw : Inport  Port=4
  TwIm : Inport  Port=5
  TwRe : Inport  Port=6
  dvld : Inport  Port=7
  syncin : Inport  Port=8
  AddSub : xbsIndex_r4/AddSub  mode=Addition  use_carryin=off  use_carryout=off  en=off  latency=1  precision=Full  arith_type=Unsigned  n_bits=16  bin_pt=14  quantization=Truncate  overflow=Wrap  dbl_ovrd=off  use_behavioral_HDL=off  hw_selection=Fabric  pipelined=off  block_type=addsub
  AddSub1 : xbsIndex_r4/AddSub  mode=Addition  use_carryin=off  use_carryout=off  en=off  latency=1  precision=Full  arith_type=Unsigned  n_bits=16  bin_pt=14  quantization=Truncate  overflow=Wrap  dbl_ovrd=off  use_behavioral_HDL=off  hw_selection=Fabric  pipelined=off  block_type=addsub
  "Complex Multiplier 5.0 " : xbsIndex_r4/Complex Multiplier 5.0   hasatlast=on  hasatuser=off  atuserwidth=1  hasbtlast=off  hasbtuser=off  btuserwidth=1  multtype=Use_Mults  optimizegoal=Resources  flowcontrol=NonBlocking  outputwidth=33  roundmode=Truncate  hasctrltlast=off  hasctrltuser=off  ctrltuserwidth=1  outtlastbehv=Pass_A_TLAST  latencyconfig=Automatic  minimumlatency=37  aclken=off  aresetn=off  trim_axipin_name=on  aportwidth=63  bportwidth=63  ip_name=Complex Multiplier  ip_version=5.0  dsptool_ready=true  ipcore_usecache=true  ipcore_useipmodelcache=true  ipcore_verbose=false  ipcore_latency_parameter='minimumlatency'  wrapper_available=true  port_translation_map={ 'aclken' => 'en', 'aresetn' => 'rst'}  structural_sim=false  block_type=cmpy_v5_0
  Complex to Magnitude-Angle{,1..5} (6 alike) : ComplexToMagnitudeAngle
  Convert{,1..7} (8 alike) : xbsIndex_r4/Convert  gui_display_data_type=Fixed-point  arith_type="Signed  (2's comp)"  n_bits=16  bin_pt=14  float_type=Single  exp_bits=8  fraction_bits=24  quantization=Truncate  overflow=Wrap  en=off  latency=0  dbl_ovrd=off  pipeline=off  block_type=convert
  Delay : xbsIndex_r4/Delay  rst=off  infoeditControl=Selection of Reset will increase slice count due to use of real FFs and instead of SRLs  en=off  latency=6  dbl_ovrd=off  reg_retiming=off  block_type=delay
  Delay1 : xbsIndex_r4/Delay  rst=off  infoeditControl=Selection of Reset will increase slice count due to use of real FFs and instead of SRLs  en=off  latency=6  dbl_ovrd=off  reg_retiming=off  block_type=delay
  Delay2 : xbsIndex_r4/Delay  rst=off  infoeditControl=Selection of Reset will increase slice count due to use of real FFs and instead of SRLs  en=off  latency=1  dbl_ovrd=off  reg_retiming=off  block_type=delay
  Delay3 : xbsIndex_r4/Delay  rst=off  infoeditControl=Selection of Reset will increase slice count due to use of real FFs and instead of SRLs  en=off  latency=1  dbl_ovrd=off  reg_retiming=off  block_type=delay
  Gateway Out{1..14} (14 alike) : xbsIndex_r4/Gateway Out  inherit_from_input=off  hdl_port=on  timing_constraint=None  locs_specified=off  LOCs={}  UseAsDAC=off  DACChannel='1'  block_type=gatewayout
  Real-Imag to Complex{,1..5} (6 alike) : RealImagToComplex
  buttscope : Scope  NumInputPorts=6
      settings: YMin=-5~-5~-5~-5~-5~-5  YMax=5~5~5~5~5~5  SaveName=ScopeData4
  buttscope1 : Scope  NumInputPorts=8
      settings: YMin=-5~-5~-5~-5~-5~-5~-5~-5  YMax=5~5~5~5~5~5~5~5  SaveName=ScopeData6
  Imut : Outport
  ReOut : Outport  Port=2
  dvldout : Outport  Port=3
  syncout : Outport  Port=4
  wires:
  ReInOne/1 -> Convert7/1
  ImInOne/1 -> Convert6/1
  AddSub/1 -> Gateway Out6/1, Imut/1
  AddSub1/1 -> Gateway Out2/1, ReOut/1
  ImInTw/1 -> Convert3/1
  ReInTw/1 -> Convert2/1
  Delay/1 -> Gateway Out7/1, AddSub/1
  Delay1/1 -> Gateway Out3/1, AddSub1/1
  TwIm/1 -> Convert4/1
  TwRe/1 -> Convert5/1
  dvld/1 -> "Complex Multiplier 5.0 "/5, "Complex Multiplier 5.0 "/1
  Convert6/1 -> Delay/1
  Convert7/1 -> Delay1/1
  Convert3/1 -> "Complex Multiplier 5.0 "/3, Gateway Out11/1
  Convert2/1 -> "Complex Multiplier 5.0 "/4, Gateway Out12/1
  Convert4/1 -> "Complex Multiplier 5.0 "/6, Gateway Out5/1
  Convert5/1 -> "Complex Multiplier 5.0 "/7, Gateway Out8/1
  Convert1/1 -> Gateway Out10/1, Gateway Out4/1, AddSub1/2
  syncin/1 -> Gateway Out14/1, "Complex Multiplier 5.0 "/2
  "Complex Multiplier 5.0 "/4 -> Convert1/1
  "Complex Multiplier 5.0 "/3 -> Convert/1
  "Complex Multiplier 5.0 "/1 -> Delay2/1
  "Complex Multiplier 5.0 "/2 -> Gateway Out13/1, Delay3/1
  Convert/1 -> Gateway Out9/1, Gateway Out1/1, AddSub/2
  Delay2/1 -> dvldout/1
  Delay3/1 -> syncout/1
  Real-Imag to Complex/1 -> Complex to Magnitude-Angle/1
  Real-Imag to Complex1/1 -> Complex to Magnitude-Angle1/1
  Real-Imag to Complex2/1 -> Complex to Magnitude-Angle2/1
  Complex to Magnitude-Angle/1 -> buttscope1/1
  Complex to Magnitude-Angle/2 -> buttscope1/2
  Complex to Magnitude-Angle1/1 -> buttscope1/3
  Complex to Magnitude-Angle1/2 -> buttscope1/4
  Complex to Magnitude-Angle2/1 -> buttscope1/5
  Complex to Magnitude-Angle2/2 -> buttscope1/6
  Gateway Out11/1 -> Real-Imag to Complex/2
  Gateway Out12/1 -> Real-Imag to Complex/1
  Gateway Out5/1 -> Real-Imag to Complex1/2
  Gateway Out8/1 -> Real-Imag to Complex1/1
  Gateway Out9/1 -> Real-Imag to Complex2/2
  Gateway Out10/1 -> Real-Imag to Complex2/1
  Gateway Out13/1 -> buttscope1/7
  Gateway Out14/1 -> buttscope1/8
  Real-Imag to Complex3/1 -> Complex to Magnitude-Angle3/1
  Real-Imag to Complex4/1 -> Complex to Magnitude-Angle4/1
  Real-Imag to Complex5/1 -> Complex to Magnitude-Angle5/1
  Gateway Out7/1 -> Real-Imag to Complex3/2
  Gateway Out3/1 -> Real-Imag to Complex3/1
  Complex to Magnitude-Angle3/1 -> buttscope/1
  Complex to Magnitude-Angle3/2 -> buttscope/2
  Gateway Out1/1 -> Real-Imag to Complex4/2
  Gateway Out4/1 -> Real-Imag to Complex4/1
  Complex to Magnitude-Angle4/1 -> buttscope/3
  Complex to Magnitude-Angle4/2 -> buttscope/4
  Gateway Out6/1 -> Real-Imag to Complex5/2
  Gateway Out2/1 -> Real-Imag to Complex5/1
  Complex to Magnitude-Angle5/1 -> buttscope/5
  Complex to Magnitude-Angle5/2 -> buttscope/6

== system tesdd/WindowAndFFT/FFT512_/FFT_DIT512_/Butterfly2 ==
  note: same delay as cmpkx mult
  ImInOne : Inport
  ReInOne : Inport  Port=2
  ImInTw : Inport  Port=3
  ReInTw : Inport  Port=4
  TwIm : Inport  Port=5
  TwRe : Inport  Port=6
  dvld : Inport  Port=7
  syncin : Inport  Port=8
  AddSub : xbsIndex_r4/AddSub  mode=Addition  use_carryin=off  use_carryout=off  en=off  latency=1  precision=Full  arith_type=Unsigned  n_bits=16  bin_pt=14  quantization=Truncate  overflow=Wrap  dbl_ovrd=off  use_behavioral_HDL=off  hw_selection=Fabric  pipelined=off  block_type=addsub
  AddSub1 : xbsIndex_r4/AddSub  mode=Addition  use_carryin=off  use_carryout=off  en=off  latency=1  precision=Full  arith_type=Unsigned  n_bits=16  bin_pt=14  quantization=Truncate  overflow=Wrap  dbl_ovrd=off  use_behavioral_HDL=off  hw_selection=Fabric  pipelined=off  block_type=addsub
  "Complex Multiplier 5.0 " : xbsIndex_r4/Complex Multiplier 5.0   hasatlast=on  hasatuser=off  atuserwidth=1  hasbtlast=off  hasbtuser=off  btuserwidth=1  multtype=Use_Mults  optimizegoal=Resources  flowcontrol=NonBlocking  outputwidth=33  roundmode=Truncate  hasctrltlast=off  hasctrltuser=off  ctrltuserwidth=1  outtlastbehv=Pass_A_TLAST  latencyconfig=Automatic  minimumlatency=37  aclken=off  aresetn=off  trim_axipin_name=on  aportwidth=63  bportwidth=63  ip_name=Complex Multiplier  ip_version=5.0  dsptool_ready=true  ipcore_usecache=true  ipcore_useipmodelcache=true  ipcore_verbose=false  ipcore_latency_parameter='minimumlatency'  wrapper_available=true  port_translation_map={ 'aclken' => 'en', 'aresetn' => 'rst'}  structural_sim=false  block_type=cmpy_v5_0
  Complex to Magnitude-Angle{,1..5} (6 alike) : ComplexToMagnitudeAngle
  Convert{,1..7} (8 alike) : xbsIndex_r4/Convert  gui_display_data_type=Fixed-point  arith_type="Signed  (2's comp)"  n_bits=16  bin_pt=14  float_type=Single  exp_bits=8  fraction_bits=24  quantization=Truncate  overflow=Wrap  en=off  latency=0  dbl_ovrd=off  pipeline=off  block_type=convert
  Delay : xbsIndex_r4/Delay  rst=off  infoeditControl=Selection of Reset will increase slice count due to use of real FFs and instead of SRLs  en=off  latency=6  dbl_ovrd=off  reg_retiming=off  block_type=delay
  Delay1 : xbsIndex_r4/Delay  rst=off  infoeditControl=Selection of Reset will increase slice count due to use of real FFs and instead of SRLs  en=off  latency=6  dbl_ovrd=off  reg_retiming=off  block_type=delay
  Delay2 : xbsIndex_r4/Delay  rst=off  infoeditControl=Selection of Reset will increase slice count due to use of real FFs and instead of SRLs  en=off  latency=1  dbl_ovrd=off  reg_retiming=off  block_type=delay
  Delay3 : xbsIndex_r4/Delay  rst=off  infoeditControl=Selection of Reset will increase slice count due to use of real FFs and instead of SRLs  en=off  latency=1  dbl_ovrd=off  reg_retiming=off  block_type=delay
  Gateway Out{1..14} (14 alike) : xbsIndex_r4/Gateway Out  inherit_from_input=off  hdl_port=on  timing_constraint=None  locs_specified=off  LOCs={}  UseAsDAC=off  DACChannel='1'  block_type=gatewayout
  Real-Imag to Complex{,1..5} (6 alike) : RealImagToComplex
  buttscope : Scope  NumInputPorts=6
      settings: YMin=-5~-5~-5~-5~-5~-5  YMax=5~5~5~5~5~5  SaveName=ScopeData4
  buttscope1 : Scope  NumInputPorts=8
      settings: YMin=-5~-5~-5~-5~-5~-5~-5~-5  YMax=5~5~5~5~5~5~5~5  SaveName=ScopeData6
  Imut : Outport
  ReOut : Outport  Port=2
  dvldout : Outport  Port=3
  syncout : Outport  Port=4
  wires:
  ReInOne/1 -> Convert7/1
  ImInOne/1 -> Convert6/1
  AddSub/1 -> Gateway Out6/1, Imut/1
  AddSub1/1 -> Gateway Out2/1, ReOut/1
  ImInTw/1 -> Convert3/1
  ReInTw/1 -> Convert2/1
  Delay/1 -> Gateway Out7/1, AddSub/1
  Delay1/1 -> Gateway Out3/1, AddSub1/1
  TwIm/1 -> Convert4/1
  TwRe/1 -> Convert5/1
  dvld/1 -> "Complex Multiplier 5.0 "/5, "Complex Multiplier 5.0 "/1
  Convert6/1 -> Delay/1
  Convert7/1 -> Delay1/1
  Convert3/1 -> "Complex Multiplier 5.0 "/3, Gateway Out11/1
  Convert2/1 -> "Complex Multiplier 5.0 "/4, Gateway Out12/1
  Convert4/1 -> "Complex Multiplier 5.0 "/6, Gateway Out5/1
  Convert5/1 -> "Complex Multiplier 5.0 "/7, Gateway Out8/1
  Convert1/1 -> Gateway Out10/1, Gateway Out4/1, AddSub1/2
  syncin/1 -> Gateway Out14/1, "Complex Multiplier 5.0 "/2
  "Complex Multiplier 5.0 "/4 -> Convert1/1
  "Complex Multiplier 5.0 "/3 -> Convert/1
  "Complex Multiplier 5.0 "/1 -> Delay2/1
  "Complex Multiplier 5.0 "/2 -> Gateway Out13/1, Delay3/1
  Convert/1 -> Gateway Out9/1, Gateway Out1/1, AddSub/2
  Delay2/1 -> dvldout/1
  Delay3/1 -> syncout/1
  Real-Imag to Complex/1 -> Complex to Magnitude-Angle/1
  Real-Imag to Complex1/1 -> Complex to Magnitude-Angle1/1
  Real-Imag to Complex2/1 -> Complex to Magnitude-Angle2/1
  Complex to Magnitude-Angle/1 -> buttscope1/1
  Complex to Magnitude-Angle/2 -> buttscope1/2
  Complex to Magnitude-Angle1/1 -> buttscope1/3
  Complex to Magnitude-Angle1/2 -> buttscope1/4
  Complex to Magnitude-Angle2/1 -> buttscope1/5
  Complex to Magnitude-Angle2/2 -> buttscope1/6
  Gateway Out11/1 -> Real-Imag to Complex/2
  Gateway Out12/1 -> Real-Imag to Complex/1
  Gateway Out5/1 -> Real-Imag to Complex1/2
  Gateway Out8/1 -> Real-Imag to Complex1/1
  Gateway Out9/1 -> Real-Imag to Complex2/2
  Gateway Out10/1 -> Real-Imag to Complex2/1
  Gateway Out13/1 -> buttscope1/7
  Gateway Out14/1 -> buttscope1/8
  Real-Imag to Complex3/1 -> Complex to Magnitude-Angle3/1
  Real-Imag to Complex4/1 -> Complex to Magnitude-Angle4/1
  Real-Imag to Complex5/1 -> Complex to Magnitude-Angle5/1
  Gateway Out7/1 -> Real-Imag to Complex3/2
  Gateway Out3/1 -> Real-Imag to Complex3/1
  Complex to Magnitude-Angle3/1 -> buttscope/1
  Complex to Magnitude-Angle3/2 -> buttscope/2
  Gateway Out1/1 -> Real-Imag to Complex4/2
  Gateway Out4/1 -> Real-Imag to Complex4/1
  Complex to Magnitude-Angle4/1 -> buttscope/3
  Complex to Magnitude-Angle4/2 -> buttscope/4
  Gateway Out6/1 -> Real-Imag to Complex5/2
  Gateway Out2/1 -> Real-Imag to Complex5/1
  Complex to Magnitude-Angle5/1 -> buttscope/5
  Complex to Magnitude-Angle5/2 -> buttscope/6

== system tesdd/WindowAndFFT/FFT512_/FFT_DIT512_/Butterfly3 ==
  note: same delay as cmpkx mult
  ImInOne : Inport
  ReInOne : Inport  Port=2
  ImInTw : Inport  Port=3
  ReInTw : Inport  Port=4
  TwIm : Inport  Port=5
  TwRe : Inport  Port=6
  dvld : Inport  Port=7
  syncin : Inport  Port=8
  AddSub : xbsIndex_r4/AddSub  mode=Addition  use_carryin=off  use_carryout=off  en=off  latency=1  precision=Full  arith_type=Unsigned  n_bits=16  bin_pt=14  quantization=Truncate  overflow=Wrap  dbl_ovrd=off  use_behavioral_HDL=off  hw_selection=Fabric  pipelined=off  block_type=addsub
  AddSub1 : xbsIndex_r4/AddSub  mode=Addition  use_carryin=off  use_carryout=off  en=off  latency=1  precision=Full  arith_type=Unsigned  n_bits=16  bin_pt=14  quantization=Truncate  overflow=Wrap  dbl_ovrd=off  use_behavioral_HDL=off  hw_selection=Fabric  pipelined=off  block_type=addsub
  "Complex Multiplier 5.0 " : xbsIndex_r4/Complex Multiplier 5.0   hasatlast=on  hasatuser=off  atuserwidth=1  hasbtlast=off  hasbtuser=off  btuserwidth=1  multtype=Use_Mults  optimizegoal=Resources  flowcontrol=NonBlocking  outputwidth=33  roundmode=Truncate  hasctrltlast=off  hasctrltuser=off  ctrltuserwidth=1  outtlastbehv=Pass_A_TLAST  latencyconfig=Automatic  minimumlatency=37  aclken=off  aresetn=off  trim_axipin_name=on  aportwidth=63  bportwidth=63  ip_name=Complex Multiplier  ip_version=5.0  dsptool_ready=true  ipcore_usecache=true  ipcore_useipmodelcache=true  ipcore_verbose=false  ipcore_latency_parameter='minimumlatency'  wrapper_available=true  port_translation_map={ 'aclken' => 'en', 'aresetn' => 'rst'}  structural_sim=false  block_type=cmpy_v5_0
  Complex to Magnitude-Angle{,1..5} (6 alike) : ComplexToMagnitudeAngle
  Convert{,1..7} (8 alike) : xbsIndex_r4/Convert  gui_display_data_type=Fixed-point  arith_type="Signed  (2's comp)"  n_bits=16  bin_pt=14  float_type=Single  exp_bits=8  fraction_bits=24  quantization=Truncate  overflow=Wrap  en=off  latency=0  dbl_ovrd=off  pipeline=off  block_type=convert
  Delay : xbsIndex_r4/Delay  rst=off  infoeditControl=Selection of Reset will increase slice count due to use of real FFs and instead of SRLs  en=off  latency=6  dbl_ovrd=off  reg_retiming=off  block_type=delay
  Delay1 : xbsIndex_r4/Delay  rst=off  infoeditControl=Selection of Reset will increase slice count due to use of real FFs and instead of SRLs  en=off  latency=6  dbl_ovrd=off  reg_retiming=off  block_type=delay
  Delay2 : xbsIndex_r4/Delay  rst=off  infoeditControl=Selection of Reset will increase slice count due to use of real FFs and instead of SRLs  en=off  latency=1  dbl_ovrd=off  reg_retiming=off  block_type=delay
  Delay3 : xbsIndex_r4/Delay  rst=off  infoeditControl=Selection of Reset will increase slice count due to use of real FFs and instead of SRLs  en=off  latency=1  dbl_ovrd=off  reg_retiming=off  block_type=delay
  Gateway Out{1..14} (14 alike) : xbsIndex_r4/Gateway Out  inherit_from_input=off  hdl_port=on  timing_constraint=None  locs_specified=off  LOCs={}  UseAsDAC=off  DACChannel='1'  block_type=gatewayout
  Real-Imag to Complex{,1..5} (6 alike) : RealImagToComplex
  buttscope : Scope  NumInputPorts=6
      settings: YMin=-5~-5~-5~-5~-5~-5  YMax=5~5~5~5~5~5  SaveName=ScopeData4
  buttscope1 : Scope  NumInputPorts=8
      settings: YMin=-5~-5~-5~-5~-5~-5~-5~-5  YMax=5~5~5~5~5~5~5~5  SaveName=ScopeData6
  Imut : Outport
  ReOut : Outport  Port=2
  dvldout : Outport  Port=3
  syncout : Outport  Port=4
  wires:
  ReInOne/1 -> Convert7/1
  ImInOne/1 -> Convert6/1
  AddSub/1 -> Gateway Out6/1, Imut/1
  AddSub1/1 -> Gateway Out2/1, ReOut/1
  ImInTw/1 -> Convert3/1
  ReInTw/1 -> Convert2/1
  Delay/1 -> Gateway Out7/1, AddSub/1
  Delay1/1 -> Gateway Out3/1, AddSub1/1
  TwIm/1 -> Convert4/1
  TwRe/1 -> Convert5/1
  dvld/1 -> "Complex Multiplier 5.0 "/5, "Complex Multiplier 5.0 "/1
  Convert6/1 -> Delay/1
  Convert7/1 -> Delay1/1
  Convert3/1 -> "Complex Multiplier 5.0 "/3, Gateway Out11/1
  Convert2/1 -> "Complex Multiplier 5.0 "/4, Gateway Out12/1
  Convert4/1 -> "Complex Multiplier 5.0 "/6, Gateway Out5/1
  Convert5/1 -> "Complex Multiplier 5.0 "/7, Gateway Out8/1
  Convert1/1 -> Gateway Out10/1, Gateway Out4/1, AddSub1/2
  syncin/1 -> Gateway Out14/1, "Complex Multiplier 5.0 "/2
  "Complex Multiplier 5.0 "/4 -> Convert1/1
  "Complex Multiplier 5.0 "/3 -> Convert/1
  "Complex Multiplier 5.0 "/1 -> Delay2/1
  "Complex Multiplier 5.0 "/2 -> Gateway Out13/1, Delay3/1
  Convert/1 -> Gateway Out9/1, Gateway Out1/1, AddSub/2
  Delay2/1 -> dvldout/1
  Delay3/1 -> syncout/1
  Real-Imag to Complex/1 -> Complex to Magnitude-Angle/1
  Real-Imag to Complex1/1 -> Complex to Magnitude-Angle1/1
  Real-Imag to Complex2/1 -> Complex to Magnitude-Angle2/1
  Complex to Magnitude-Angle/1 -> buttscope1/1
  Complex to Magnitude-Angle/2 -> buttscope1/2
  Complex to Magnitude-Angle1/1 -> buttscope1/3
  Complex to Magnitude-Angle1/2 -> buttscope1/4
  Complex to Magnitude-Angle2/1 -> buttscope1/5
  Complex to Magnitude-Angle2/2 -> buttscope1/6
  Gateway Out11/1 -> Real-Imag to Complex/2
  Gateway Out12/1 -> Real-Imag to Complex/1
  Gateway Out5/1 -> Real-Imag to Complex1/2
  Gateway Out8/1 -> Real-Imag to Complex1/1
  Gateway Out9/1 -> Real-Imag to Complex2/2
  Gateway Out10/1 -> Real-Imag to Complex2/1
  Gateway Out13/1 -> buttscope1/7
  Gateway Out14/1 -> buttscope1/8
  Real-Imag to Complex3/1 -> Complex to Magnitude-Angle3/1
  Real-Imag to Complex4/1 -> Complex to Magnitude-Angle4/1
  Real-Imag to Complex5/1 -> Complex to Magnitude-Angle5/1
  Gateway Out7/1 -> Real-Imag to Complex3/2
  Gateway Out3/1 -> Real-Imag to Complex3/1
  Complex to Magnitude-Angle3/1 -> buttscope/1
  Complex to Magnitude-Angle3/2 -> buttscope/2
  Gateway Out1/1 -> Real-Imag to Complex4/2
  Gateway Out4/1 -> Real-Imag to Complex4/1
  Complex to Magnitude-Angle4/1 -> buttscope/3
  Complex to Magnitude-Angle4/2 -> buttscope/4
  Gateway Out6/1 -> Real-Imag to Complex5/2
  Gateway Out2/1 -> Real-Imag to Complex5/1
  Complex to Magnitude-Angle5/1 -> buttscope/5
  Complex to Magnitude-Angle5/2 -> buttscope/6
